simulink model "PassStCaller"  (R2018b)
settings: Solver=FixedStepDiscrete  StartTime=0.0  StopTime=10.0  FixedStep=0.01  RelTol=1e-3
undefined symbols (not defined in the file or in its folder): PassStBkReclnCtrl_1_Cal, PassStBkReclnHolderChk_1_Cal, PassStBkReclnIsPosChk_1_Cal, PassStBkReclnTrgtPosSelc_1_Cal, PassStCshnFldCtrl_1_Cal, PassStCshnFldHolderChk_1_Cal, PassStCshnFldIsPosChk_1_Cal, PassStCshnFldTrgtPosSelc_1_Cal, PassStFtCtrl_1_Cal, PassStFtHolderChk_1_Cal, PassStFtIsPosChk_1_Cal, PassStFtTrgtPosSelc_1_Cal, PassStFwdbkwdCtrl_1_Cal, PassStFwdBkwdHolderChk_1_Cal, PassStFwdBkwdIsPosChk_1_Cal, PassStFwdBkwdTrgtPosSelc_1_Cal, PassStRclCmdSrvCal_1_Cal
settings Model: ModifiedHistory=V3.0.0 557模式流程V1.9  Creator=sn2xws  LastModifiedBy=sn2xws
settings DataIOCC: SaveFormat=StructureWithTime
settings OptimizationCC: DefaultParameterBehavior=Inlined  EnhancedBackFolding=on  PassReuseOutputArgsAs=Individual arguments  ZeroExternalMemoryAtStartup=off  ZeroInternalMemoryAtStartup=off  OptimizeBlockOrder=speed  DifferentSizesBufferReuse=on  OptimizationCustomize=off
settings DebuggingCC: ParameterTunabilityLossMsg=error
settings SFSimCC: MATLABDynamicMemAlloc=off
settings RTWCC: SystemTargetFile=autosar.tlc  GenCodeOnly=on  TemplateMakefile=ert_default_tmf  Description=AUTOSAR  GenerateReport=on  IncludeHyperlinkInReport=on  LaunchReport=on  GenerateTraceInfo=on  GenerateTraceReport=on  GenerateTraceReportSl=on  GenerateTraceReportSf=on  GenerateTraceReportEml=on
settings CodeAppCC: ForceParamTrailComments=on  IgnoreCustomStorageClasses=off  OperatorAnnotations=on  SimulinkDataObjDesc=on  SFDataObjDesc=on  InsertBlockDesc=on
settings STFCustomTargetCC: TargetLangStandard=C99 (ISO)  MultiwordLength=256  ParMdlRefBuildCompliant=on  CompOptLevelCompliant=on  IncludeMdlTerminateFcn=off  CombineOutputUpdateFcns=on  SuppressErrorStatus=on  ERTCustomFileBanners=on  SupportNonFinite=off  SupportComplex=off  SupportContinuousTime=off  SupportNonInlinedSFcns=off  RemoveResetFunc=on  MATLABClassNameForMDSCustomization=Simulink.SoftwareTarget.ERTCustomization  AutosarCompliant=on  UseToolchainInfoCompliant=on  LookupTableObjectStructAxisOrder=2,1,3,4,...  LUTObjectStructOrderEvenSpacing=Size,Table,Breakpoints  SystemTargetFile=autosar.tlc
settings ERTTargetCC: TargetLangStandard=C99 (ISO)  ConcurrentExecutionCompliant=off  IncludeMdlTerminateFcn=off  SuppressErrorStatus=on  SupportNonFinite=off  SupportComplex=off  ModelStepFunctionPrototypeControlCompliant=off  CPPClassGenCompliant=off  AutosarCompliant=on  LookupTableObjectStructAxisOrder=2,1,3,4,...  LUTObjectStructOrderEvenSpacing=Size,Table,Breakpoints  InlinedParameterPlacement=NonHierarchical  ERTCustomFileTemplate=example_file_process.tlc  ERTFilePackagingFormat=Compact

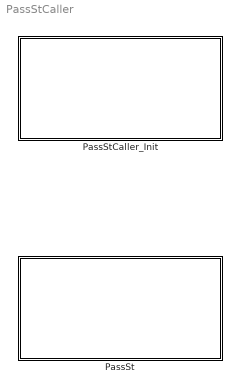
== system PassStCaller ==
  PassSt : Subsystem
  PassStCaller_Init : Subsystem

== system PassStCaller/PassSt ==
  PassSt_Cal_sys : Subsystem

== system PassStCaller/PassStCaller_Init ==
  Event Listener : EventListener  EventName=reset

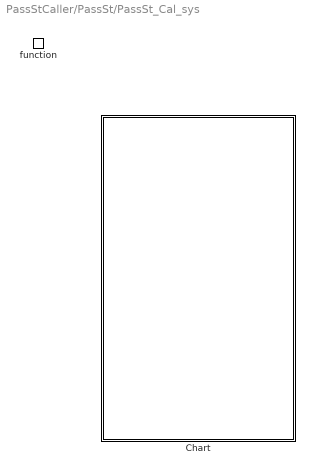
== system PassStCaller/PassSt/PassSt_Cal_sys ==
  function : TriggerPort  TriggerType=function-call  IsSimulinkFunction=on  FunctionName=PassSt_Cal  VariantControl=(inherit)
  Chart : Stateflow chart  TreatAsAtomicUnit=on

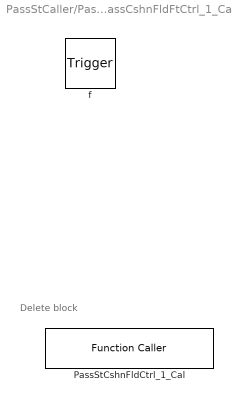
== system PassStCaller/PassSt/PassSt_Cal_sys/Chart/PassCshnFldFtCtrl_1_Cal ==
  note: Delete block
  f : TriggerPort  TriggerType=function-call  VariantControl=(inherit)
      settings: CopyFcn=Stateflow.SLINSF.SimulinkMan.removeBlockPreDeleteFcn  PreDeleteFcn=Stateflow.SLINSF.SimulinkMan.unsafePredeleteFcn
  PassStCshnFldCtrl_1_Cal : FunctionCaller  FunctionPrototype=PassStCshnFldCtrl_1_Cal()

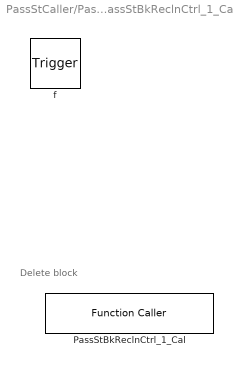
== system PassStCaller/PassSt/PassSt_Cal_sys/Chart/PassStBkReclnCtrl_1_Cal ==
  note: Delete block
  f : TriggerPort  TriggerType=function-call  VariantControl=(inherit)
      settings: CopyFcn=Stateflow.SLINSF.SimulinkMan.removeBlockPreDeleteFcn  PreDeleteFcn=Stateflow.SLINSF.SimulinkMan.unsafePredeleteFcn
  PassStBkReclnCtrl_1_Cal : FunctionCaller  FunctionPrototype=PassStBkReclnCtrl_1_Cal()

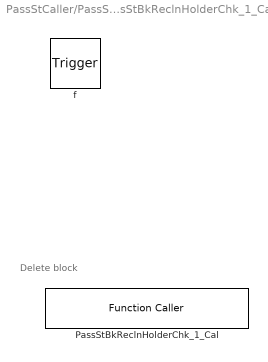
== system PassStCaller/PassSt/PassSt_Cal_sys/Chart/PassStBkReclnHolderChk_1_Cal ==
  note: Delete block
  f : TriggerPort  TriggerType=function-call  VariantControl=(inherit)
      settings: CopyFcn=Stateflow.SLINSF.SimulinkMan.removeBlockPreDeleteFcn  PreDeleteFcn=Stateflow.SLINSF.SimulinkMan.unsafePredeleteFcn
  PassStBkReclnHolderChk_1_Cal : FunctionCaller  FunctionPrototype=PassStBkReclnHolderChk_1_Cal()

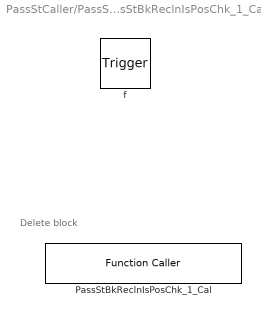
== system PassStCaller/PassSt/PassSt_Cal_sys/Chart/PassStBkReclnIsPosChk_1_Cal ==
  note: Delete block
  f : TriggerPort  TriggerType=function-call  VariantControl=(inherit)
      settings: CopyFcn=Stateflow.SLINSF.SimulinkMan.removeBlockPreDeleteFcn  PreDeleteFcn=Stateflow.SLINSF.SimulinkMan.unsafePredeleteFcn
  PassStBkReclnIsPosChk_1_Cal : FunctionCaller  FunctionPrototype=PassStBkReclnIsPosChk_1_Cal()

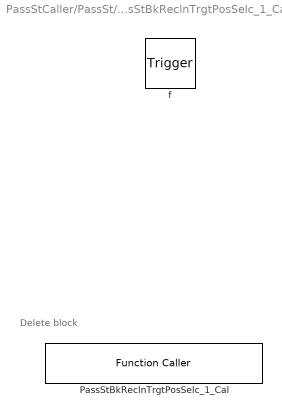
== system PassStCaller/PassSt/PassSt_Cal_sys/Chart/PassStBkReclnTrgtPosSelc_1_Cal ==
  note: Delete block
  f : TriggerPort  TriggerType=function-call  VariantControl=(inherit)
      settings: CopyFcn=Stateflow.SLINSF.SimulinkMan.removeBlockPreDeleteFcn  PreDeleteFcn=Stateflow.SLINSF.SimulinkMan.unsafePredeleteFcn
  PassStBkReclnTrgtPosSelc_1_Cal : FunctionCaller  FunctionPrototype=PassStBkReclnTrgtPosSelc_1_Cal()

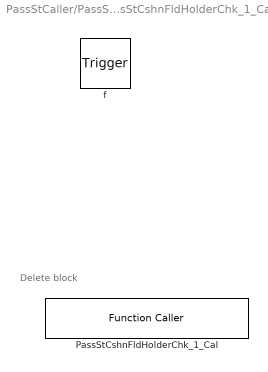
== system PassStCaller/PassSt/PassSt_Cal_sys/Chart/PassStCshnFldHolderChk_1_Cal ==
  note: Delete block
  f : TriggerPort  TriggerType=function-call  VariantControl=(inherit)
      settings: CopyFcn=Stateflow.SLINSF.SimulinkMan.removeBlockPreDeleteFcn  PreDeleteFcn=Stateflow.SLINSF.SimulinkMan.unsafePredeleteFcn
  PassStCshnFldHolderChk_1_Cal : FunctionCaller  FunctionPrototype=PassStCshnFldHolderChk_1_Cal()

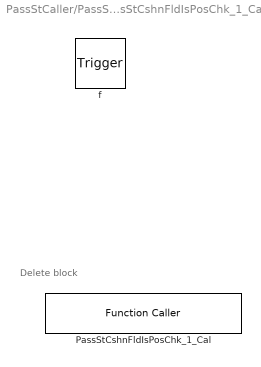
== system PassStCaller/PassSt/PassSt_Cal_sys/Chart/PassStCshnFldIsPosChk_1_Cal ==
  note: Delete block
  f : TriggerPort  TriggerType=function-call  VariantControl=(inherit)
      settings: CopyFcn=Stateflow.SLINSF.SimulinkMan.removeBlockPreDeleteFcn  PreDeleteFcn=Stateflow.SLINSF.SimulinkMan.unsafePredeleteFcn
  PassStCshnFldIsPosChk_1_Cal : FunctionCaller  FunctionPrototype=PassStCshnFldIsPosChk_1_Cal()

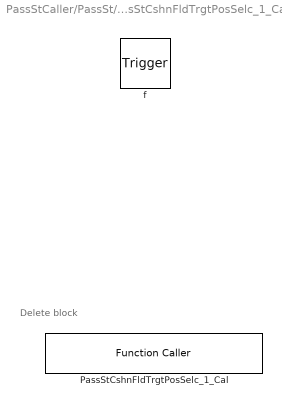
== system PassStCaller/PassSt/PassSt_Cal_sys/Chart/PassStCshnFldTrgtPosSelc_1_Cal ==
  note: Delete block
  f : TriggerPort  TriggerType=function-call  VariantControl=(inherit)
      settings: CopyFcn=Stateflow.SLINSF.SimulinkMan.removeBlockPreDeleteFcn  PreDeleteFcn=Stateflow.SLINSF.SimulinkMan.unsafePredeleteFcn
  PassStCshnFldTrgtPosSelc_1_Cal : FunctionCaller  FunctionPrototype=PassStCshnFldTrgtPosSelc_1_Cal()

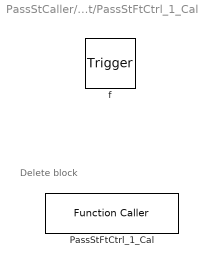
== system PassStCaller/PassSt/PassSt_Cal_sys/Chart/PassStFtCtrl_1_Cal ==
  note: Delete block
  f : TriggerPort  TriggerType=function-call  VariantControl=(inherit)
      settings: CopyFcn=Stateflow.SLINSF.SimulinkMan.removeBlockPreDeleteFcn  PreDeleteFcn=Stateflow.SLINSF.SimulinkMan.unsafePredeleteFcn
  PassStFtCtrl_1_Cal : FunctionCaller  FunctionPrototype=PassStFtCtrl_1_Cal()

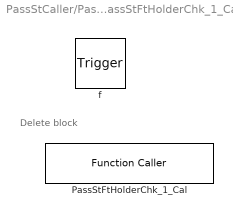
== system PassStCaller/PassSt/PassSt_Cal_sys/Chart/PassStFtHolderChk_1_Cal ==
  note: Delete block
  f : TriggerPort  TriggerType=function-call  VariantControl=(inherit)
      settings: CopyFcn=Stateflow.SLINSF.SimulinkMan.removeBlockPreDeleteFcn  PreDeleteFcn=Stateflow.SLINSF.SimulinkMan.unsafePredeleteFcn
  PassStFtHolderChk_1_Cal : FunctionCaller  FunctionPrototype=PassStFtHolderChk_1_Cal()

== system PassStCaller/PassSt/PassSt_Cal_sys/Chart/PassStFtIsPosChk_1_Cal ==
  note: Delete block
  f : TriggerPort  TriggerType=function-call  VariantControl=(inherit)
      settings: CopyFcn=Stateflow.SLINSF.SimulinkMan.removeBlockPreDeleteFcn  PreDeleteFcn=Stateflow.SLINSF.SimulinkMan.unsafePredeleteFcn
  PassStFtIsPosChk_1_Cal : FunctionCaller  FunctionPrototype=PassStFtIsPosChk_1_Cal()

== system PassStCaller/PassSt/PassSt_Cal_sys/Chart/PassStFtTrgtPosSelc_1_Cal ==
  note: Delete block
  f : TriggerPort  TriggerType=function-call  VariantControl=(inherit)
      settings: CopyFcn=Stateflow.SLINSF.SimulinkMan.removeBlockPreDeleteFcn  PreDeleteFcn=Stateflow.SLINSF.SimulinkMan.unsafePredeleteFcn
  PassStFtTrgtPosSelc_1_Cal : FunctionCaller  FunctionPrototype=PassStFtTrgtPosSelc_1_Cal()

== system PassStCaller/PassSt/PassSt_Cal_sys/Chart/PassStFwdBkwdCtrl_1_Cal ==
  note: Delete block
  f : TriggerPort  TriggerType=function-call  VariantControl=(inherit)
      settings: CopyFcn=Stateflow.SLINSF.SimulinkMan.removeBlockPreDeleteFcn  PreDeleteFcn=Stateflow.SLINSF.SimulinkMan.unsafePredeleteFcn
  PassStFwdbkwdCtrl_1_Cal : FunctionCaller  FunctionPrototype=PassStFwdbkwdCtrl_1_Cal()

== system PassStCaller/PassSt/PassSt_Cal_sys/Chart/PassStFwdBkwdHolderChk_1_Cal ==
  note: Delete block
  f : TriggerPort  TriggerType=function-call  VariantControl=(inherit)
      settings: CopyFcn=Stateflow.SLINSF.SimulinkMan.removeBlockPreDeleteFcn  PreDeleteFcn=Stateflow.SLINSF.SimulinkMan.unsafePredeleteFcn
  PassStFwdBkwdHolderChk_1_Cal : FunctionCaller  FunctionPrototype=PassStFwdBkwdHolderChk_1_Cal()

== system PassStCaller/PassSt/PassSt_Cal_sys/Chart/PassStFwdBkwdIsPosChk_1_Cal ==
  note: Delete block
  f : TriggerPort  TriggerType=function-call  VariantControl=(inherit)
      settings: CopyFcn=Stateflow.SLINSF.SimulinkMan.removeBlockPreDeleteFcn  PreDeleteFcn=Stateflow.SLINSF.SimulinkMan.unsafePredeleteFcn
  PassStFwdBkwdIsPosChk_1_Cal : FunctionCaller  FunctionPrototype=PassStFwdBkwdIsPosChk_1_Cal()

== system PassStCaller/PassSt/PassSt_Cal_sys/Chart/PassStFwdBkwdTrgtPosSelc_1_Cal ==
  note: Delete block
  f : TriggerPort  TriggerType=function-call  VariantControl=(inherit)
      settings: CopyFcn=Stateflow.SLINSF.SimulinkMan.removeBlockPreDeleteFcn  PreDeleteFcn=Stateflow.SLINSF.SimulinkMan.unsafePredeleteFcn
  PassStFwdBkwdTrgtPosSelc_1_Cal : FunctionCaller  FunctionPrototype=PassStFwdBkwdTrgtPosSelc_1_Cal()

== system PassStCaller/PassSt/PassSt_Cal_sys/Chart/PassStRclCmdSrvCal_1_Cal ==
  note: Delete block
  f : TriggerPort  TriggerType=function-call  VariantControl=(inherit)
      settings: CopyFcn=Stateflow.SLINSF.SimulinkMan.removeBlockPreDeleteFcn  PreDeleteFcn=Stateflow.SLINSF.SimulinkMan.unsafePredeleteFcn
  PassStRclCmdSrvCal_1_Cal : FunctionCaller  FunctionPrototype=PassStRclCmdSrvCal_1_Cal()

== stateflow chart PassStCaller/PassSt/PassSt_Cal_sys/Chart ==
  state PassStFtTrgtPosSelc_1_Cal [function]
  state PassStFwdBkwdTrgtPosSelc_1_Cal [function]
  state PassStCshnFldTrgtPosSelc_1_Cal [function]
  state PassStBkReclnTrgtPosSelc_1_Cal [function]
  state PassStFtIsPosChk_1_Cal [function]
  state PassStFwdBkwdIsPosChk_1_Cal [function]
  state PassStCshnFldIsPosChk_1_Cal [function]
  state PassStBkReclnIsPosChk_1_Cal [function]
  state PassStFtHolderChk_1_Cal [function]
  state PassStFwdBkwdHolderChk_1_Cal [function]
  state PassStCshnFldHolderChk_1_Cal [function]
  state PassStBkReclnHolderChk_1_Cal [function]
  state PassStFtCtrl_1_Cal [function]
  state PassStFwdBkwdCtrl_1_Cal [function]
  state PassCshnFldFtCtrl_1_Cal [function]
  state PassStBkReclnCtrl_1_Cal [function]
  state PassStRclCmdSrvCal_1_Cal [function]
  (default) -> (junction 1)
  (junction 1) -> (junction 3) : {
      | PassStFtTrgtPosSelc_1_Cal();
      | PassStFtIsPosChk_1_Cal();
      | PassStFtHolderChk_1_Cal();
      | PassStFtCtrl_1_Cal();
      | PassStFwdBkwdTrgtPosSelc_1_Cal();
      | PassStFwdBkwdIsPosChk_1_Cal();
      | PassStFwdBkwdHolderChk_1_Cal();
      | PassStFwdBkwdCtrl_1_Cal();
      | PassStCshnFldTrgtPosSelc_1_Cal();
      | PassStCshnFldIsPosChk_1_Cal();
      | PassStCshnFldHolderChk_1_Cal();
      | PassCshnFldFtCtrl_1_Cal();
      | PassStBkReclnTrgtPosSelc_1_Cal();
      | PassStBkReclnIsPosChk_1_Cal();
      | PassStBkReclnHolderChk_1_Cal();
      | PassStBkReclnCtrl_1_Cal();
      | PassStRclCmdSrvCal_1_Cal();
      | }
